simulink model "pendu_vesc_modified"  (R2020a)
settings: Solver=FixedStepAuto  StartTime=0.0  StopTime=inf  RelTol=1e-3  EnableMultiTasking=on
model workspace (MAT data in the model file):
  Da = 2
  Du = 1
  H = 60
  J = 1
  K = 1
  M : object (value not decoded)
  N = 20
  S0 = [0.01 0 0 0 0 0.01 0 0 0 0 0.0001 0 ... (16 elements, 4x4)]
  S0Sim = [0.01 0 0 0 0 0.01 0 0 0 0 0.0001 0 ... (16 elements, 4x4)]
  Sig : Simulink.Signal (value not decoded)
  Sig1 : Simulink.Signal (value not decoded)
  Sigma : object (value not decoded)
  T = 3
  Xh = [3.23195665748 2.09576255698 -0.136551314425 -0.588254405024 -0.201907649817 2.18567618171 -3.25197677698 1.14254532077 -1.68859776393 2.3666318046 2.42554352774 0.153414508771 ... (36 elements, 9x4)]
  angi = [3 4]
  augi = []
  basename = 'pendubot_'
  cc = [0 0 -9.9995000125e-05 0 0 0 -1.22458556834e-20 0 0 0 0 -9.9995000125e-05 ... (16 elements, 4x4)]
  cost : object (value not decoded)
  difi = [1 2 3 4]
  dt = 0.05
  dyni = [1 2 5 6 7 8]
  dynmodel : object (value not decoded)
  dyno = [1 2 3 4]
  fX3 = [57.5848751283 57.5848706735 57.584870567 57.5848705445 57.584869604 57.5848692003 57.5848690287 57.584868717 57.5848685976 57.5848685293 57.5848683991 57.5848682957 ... (151 elements, 151x1)]
  fantasy : object (value not decoded)
  i = 108
  j = 1
  mm = [0; 0; 3.14159265359; 3.14159265359; 1.22458556834e-16; -0.99995000125; 1.22458556834e-16; -0.99995000125]
  mu0 = [0; 0; 3.14159265359; 3.14159265359]
  mu0Sim = [0; 0; 3.14159265359; 3.14159265359]
  nc = 200
  odei = [1 2 3 4]
  opt : object (value not decoded)
  plant : object (value not decoded)
  plotting : verbosity (value not decoded)
  poli = [1 2 5 6 7 8]
  policy : object (value not decoded)
  rd = '../../'
  realCost : object (value not decoded)
  record_data = [3.14159265359 -3.1396751776 0.0306796157577 0 0 3.14159265359 -3.1408256632 -0.0230097118183 0 0.0167798938511 3.14159265359 3.14120915839 ... (545 elements, 5x109)]
  s = [3.99154064865; -6.40884909322; 3.07813248092; -2.1607954049; 0.0634175868444; -0.997987078914; -0.830941192004; -0.556360256876]
  sa = [0.0634175868444; -0.997987078914; -0.830941192004; -0.556360256876]
  ss = [0.01 0 0 0 0 0 0 0 0 0.01 0 0 ... (64 elements, 8x8)]
  trainOpt = [200 200]
  x = [0.0306796157577 -0.0230097118183 -0.0230097118183 -0.27412822575 0.0873506184902 1.75503381101 1.22816627149 -0.676608032868 -1.33717744439 -2.33662132144 -2.60950904676 -2.36326465025 ... (972 elements, 108x9)]
  x_ = [3.14159265359 3.14159265359 3.14159265359 -3.11771653557 -3.0819023985 -3.13719441642 3.01718558664 2.86638914992 2.73318560862 2.6734953269 2.7155927132 2.87392898507 ... (540 elements, 108x5)]
  xaug = [0.0306796157577 -0.0230097118183 -0.0230097118183 -0.27412822575 0.0873506184902 1.75503381101 1.22816627149 -0.676608032868 -1.33717744439 -2.33662132144 -2.60950904676 -2.36326465025 ... (864 elements, 108x8)]
  y = [-0.0230097118183 -0.0230097118183 -0.27412822575 0.0873506184902 1.75503381101 1.22816627149 -0.676608032868 -1.33717744439 -2.33662132144 -2.60950904676 -2.36326465025 -0.567289531178 ... (432 elements, 108x4)]
  y_ = [3.14159265359 3.14159265359 -3.11771653557 -3.0819023985 -3.13719441642 3.01718558664 2.86638914992 2.73318560862 2.6734953269 2.7155927132 2.87392898507 3.11017672705 ... (432 elements, 108x4)]
undefined symbols (not defined in the file or in its folder): DiscIntNeverNeededParam
libraries: eeGeneralControl x3, cm_custom x2, simulink x1
(part 2 of 2)

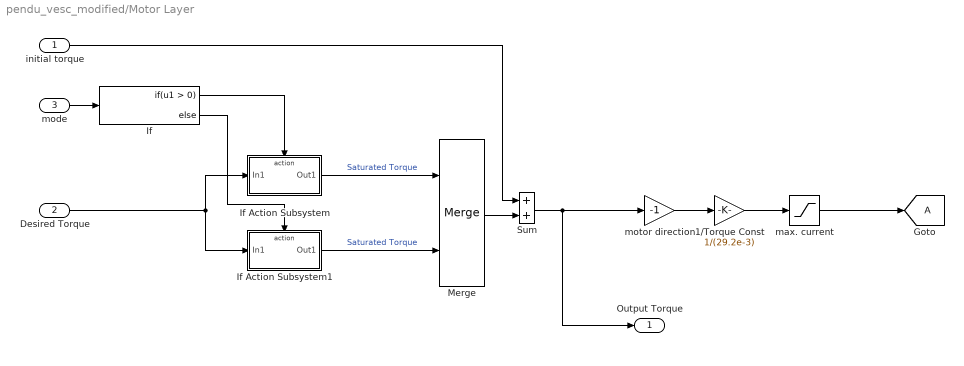
== system pendu_vesc_modified/Motor Layer ==
  initial torque : Inport
  Desired Torque : Inport  Port=2
  " mode " : Inport  Port=3
  1/Torque Const : Gain  Gain=1/(29.2e-3)  OutDataTypeStr=Inherit: Same as input
  If : If
  If Action Subsystem : Subsystem  TreatAsAtomicUnit=on
  If Action Subsystem1 : Subsystem  TreatAsAtomicUnit=on
  Merge : Merge
  Sum : Sum
  max. current : Saturate  UpperLimit=3  LowerLimit=-3  LinearizeAsGain=off
  motor direction : Gain  Gain=-1  OutDataTypeStr=Inherit: Same as input
  Output Torque : Outport  VectorParamsAs1DForOutWhenUnconnected=off
  tag scope: A=global
  wires:
  motor direction/1 -> 1/Torque Const/1
  1/Torque Const/1 -> max. current/1
  max. current/1 -> [A]
  " mode "/1 -> If/1
  Desired Torque/1 -> If Action Subsystem/1(In1), If Action Subsystem1/1(In1)
  If Action Subsystem/1(Out1) -> Merge/1  "Saturated Torque"
  If Action Subsystem1/1(Out1) -> Merge/2  "Saturated Torque"
  If/1 -> If Action Subsystem/Action
  If/2 -> If Action Subsystem1/Action
  Merge/1 -> Sum/2
  Sum/1 -> Output Torque/1, motor direction/1
  initial torque/1 -> Sum/1

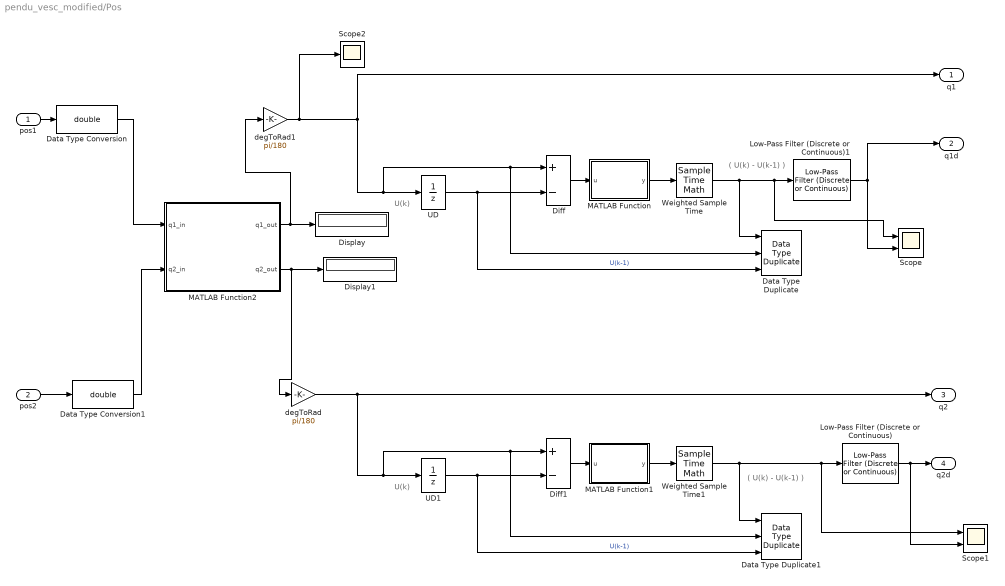
== system pendu_vesc_modified/Pos ==
  note: ( U(k) - U(k-1) )
  note: U(k)
  note: U(k)
  note: ( U(k) - U(k-1) )
  pos1 : Inport
  pos2 : Inport  Port=2
  Data Type Duplicate : DataTypeDuplicate  DisableCoverage=on  NumInputPorts=3
  Data Type Duplicate1 : DataTypeDuplicate  DisableCoverage=on  NumInputPorts=3
  Data Type Conversion : DataTypeConversion  OutDataTypeStr=double
  Data Type Conversion1 : DataTypeConversion  OutDataTypeStr=double
  Diff : Sum  Description=Add in CPU  Inputs=+-
  Diff1 : Sum  Description=Add in CPU  Inputs=+-
  Display : Display
  Display1 : Display
  Low-Pass Filter (Discrete or Continuous) : eeGeneralControl/Low-Pass Filter (Discrete or Continuous)  K=1  T=0.01  B=inf  A=-inf  init_option=Inherited from block input  x0=0  Ts=-1
  Low-Pass Filter (Discrete or Continuous)1 : eeGeneralControl/Low-Pass Filter (Discrete or Continuous)  K=1  T=0.01  B=inf  A=-inf  init_option=Inherited from block input  x0=0  Ts=-1
  MATLAB Function : MATLAB Function  TreatAsAtomicUnit=on
  MATLAB Function1 : MATLAB Function  TreatAsAtomicUnit=on
  MATLAB Function2 : MATLAB Function  TreatAsAtomicUnit=on
  Scope : Scope  NumInputPorts=2
  Scope1 : Scope  NumInputPorts=2
  Scope2 : Scope
  UD : UnitDelay  Description=Store in Global RAM  DisableCoverage=on  SampleTime=-1  HasFrameUpgradeWarning=on
  UD1 : UnitDelay  Description=Store in Global RAM  DisableCoverage=on  SampleTime=-1  HasFrameUpgradeWarning=on
  Weighted Sample Time : SampleTimeMath  TsampMathOp=/
  Weighted Sample Time1 : SampleTimeMath  TsampMathOp=/
  degToRad : Gain  Gain=pi/180
  degToRad1 : Gain  Gain=pi/180
  q1 : Outport  VectorParamsAs1DForOutWhenUnconnected=off
  q1d : Outport  Port=2  VectorParamsAs1DForOutWhenUnconnected=off
  q2 : Outport  Port=3  VectorParamsAs1DForOutWhenUnconnected=off
  q2d : Outport  Port=4  VectorParamsAs1DForOutWhenUnconnected=off
  wires:
  pos2/1 -> Data Type Conversion1/1
  pos1/1 -> Data Type Conversion/1
  Diff/1 -> MATLAB Function/1(u)
  UD/1 -> Diff/2, Data Type Duplicate/3  "U(k-1)"
  MATLAB Function/1(y) -> Weighted Sample Time/1
  Weighted Sample Time/1 -> Data Type Duplicate/1, Scope/1, Low-Pass Filter (Discrete or Continuous)1/1
  UD1/1 -> Diff1/2, Data Type Duplicate1/3  "U(k-1)"
  Diff1/1 -> MATLAB Function1/1(u)
  MATLAB Function1/1(y) -> Weighted Sample Time1/1
  Weighted Sample Time1/1 -> Data Type Duplicate1/1, Scope1/1, Low-Pass Filter (Discrete or Continuous)/1
  degToRad1/1 -> Scope2/1, q1/1, UD/1, Diff/1, Data Type Duplicate/2
  Low-Pass Filter (Discrete or Continuous)/1 -> Scope1/2, q2d/1
  Low-Pass Filter (Discrete or Continuous)1/1 -> Scope/2, q1d/1
  degToRad/1 -> q2/1, UD1/1, Diff1/1, Data Type Duplicate1/2
  Data Type Conversion/1 -> MATLAB Function2/1(q1_in)
  Data Type Conversion1/1 -> MATLAB Function2/2(q2_in)
  MATLAB Function2/1(q1_out) -> Display/1, degToRad1/1
  MATLAB Function2/2(q2_out) -> Display1/1, degToRad/1

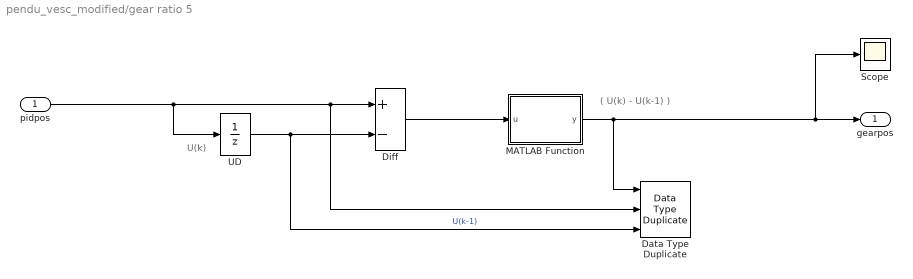
== system pendu_vesc_modified/gear ratio 5 ==
  note: ( U(k) - U(k-1) )
  note: U(k)
  pidpos : Inport
  Data Type Duplicate : DataTypeDuplicate  DisableCoverage=on  NumInputPorts=3
  Diff : Sum  Description=Add in CPU  Inputs=+-
  MATLAB Function : MATLAB Function  TreatAsAtomicUnit=on
  Scope : Scope
  UD : UnitDelay  Description=Store in Global RAM  DisableCoverage=on  SampleTime=-1  HasFrameUpgradeWarning=on
  gearpos : Outport  VectorParamsAs1DForOutWhenUnconnected=off
  wires:
  UD/1 -> Diff/2, Data Type Duplicate/3  "U(k-1)"
  pidpos/1 -> UD/1, Diff/1, Data Type Duplicate/2
  MATLAB Function/1(y) -> Data Type Duplicate/1, Scope/1, gearpos/1
  Diff/1 -> MATLAB Function/1(u)

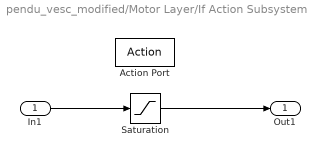
== system pendu_vesc_modified/Motor Layer/If Action Subsystem ==
  In1 : Inport
  Action Port : ActionPort  ActionPortLabel=if(u1 > 0)
  Saturation : Saturate  UpperLimit=0.035  LowerLimit=-0.035
  Out1 : Outport  VectorParamsAs1DForOutWhenUnconnected=off
  wires:
  In1/1 -> Saturation/1
  Saturation/1 -> Out1/1

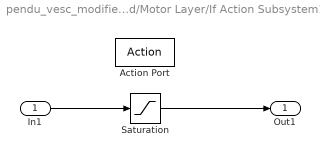
== system pendu_vesc_modified/Motor Layer/If Action Subsystem1 ==
  In1 : Inport
  Action Port : ActionPort  ActionPortLabel=else
  Saturation : Saturate  UpperLimit=0.035  LowerLimit=-0.035
  Out1 : Outport  VectorParamsAs1DForOutWhenUnconnected=off
  wires:
  In1/1 -> Saturation/1
  Saturation/1 -> Out1/1

== matlab function pendu_vesc_modified/MATLAB Function ==
  data: setzero input; u input; y output
function y = fcn(setzero,u)

persistent initpos
if isempty(initpos)
    initpos = 0;
end

if setzero
    initpos = u + 0;
end


y = u - initpos;
y = y - 360*floor(y/360);

== matlab function pendu_vesc_modified/ApplyPolicy ==
  data: x1 input size=1; tau1 output size=1; x2 input size=1; dx1 input size=1; dx2 input size=1; tau2 output size=1; mode output size=1; t input size=1; maxU input size=1; isRandPolicy input size=1; isEmptyPolicy output
function [tau1,tau2, mode, isEmptyPolicy] = ApplyPolicy(x1,x2,dx1,dx2,t,maxU, isRandPolicy)
    % % start, policy, H, plant, cost
    % angi = [3,4]

    % 
    % % % 1. Apply policy ... or random actions --------------------------------------
    % % if policy.isRandom
    % %     u = policy.fcn(policy,s(poli),zeros(length(poli)));
    % % else
    % 
    persistent policy

    if isempty(policy)
        isEmptyPolicy = 1;
        s = coder.load('pilco_load_param.mat');
        policy = s.policy;
    else
        isEmptyPolicy = 0;
    end

    u = 0;
%     persistent policy
    


    % u = maxU*(2*rand(1,1)-1);
    w = 10;
    if isRandPolicy
        u = maxU*sin(t*w);
    else

        angi = [3,4];
        poli = [1,2,5,6,7,8];
        s = [dx1, dx2, x1, x2].';
        sa = gTrig(s, zeros(length(s)), angi);
        s = [s; sa];
        mean = s(poli);
        variance = zeros(length(poli));
        hyp = policy.p.hyp;
        inputs = policy.p.inputs ;
        targets = policy.p.targets;
        u = policy_predict(hyp, inputs, targets, mean,variance, maxU) 
    end
    % % end
        tau1 = u;
        tau2 = 0;
        mode = 0;
end

== matlab function pendu_vesc_modified/MATLAB Function1 ==
  data: setzero input; u input; y output
function y = fcn(setzero,u)

persistent initpos
if isempty(initpos)
    initpos = 0;
end

if setzero
    initpos = u + 0;
end


y = u - initpos;
%y = y - 360*floor(y/360);

== matlab function pendu_vesc_modified/Pos/MATLAB Function ==
  data: u input; y output
function y = fcn(u)

u_rev = (u >= 0)*(2*pi - u) + (u < 0)*(2*pi + u);

if abs(u_rev) > abs(u)
   y = u;
else
   y = (u < 0)*u_rev - (u >= 0)*u_rev;
end

== matlab function pendu_vesc_modified/Pos/MATLAB Function1 ==
  data: u input; y output
function y = fcn(u)

u_rev = (u >= 0)*(2*pi - u) + (u < 0)*(2*pi + u);

if abs(u_rev) > abs(u)
   y = u;
else
   y = (u < 0)*u_rev - (u >= 0)*u_rev;
end

== matlab function pendu_vesc_modified/gear ratio 5/MATLAB Function ==
  data: u input; y output
function y = fcn(u)

persistent pos1
if isempty(pos1)
    pos1 = 0;
end

u_rev = (u >= 0)*(360 - u) + (u < 0)*(360 + u);
if abs(u_rev) < abs(u)
   u = (u < 0)*u_rev - (u >= 0)*u_rev;
end

u = u/5;
pos1 = pos1 + u;
pos1 = mod((pos1),360);
y = pos1;

end

== matlab function pendu_vesc_modified/Pos/MATLAB Function2 ==
  data: q1_in input; q1_out output; q2_in input; q2_out output
function [q1_out, q2_out] = convert_to_absolute(q1_in,q2_in)

q1_out = q1_in -180;

q2_out = mod(q2_in+q1_in, 360)-180;

% toggle directions
q1_out = - q1_out;
q2_out = - q2_out;
end
